simulink model "Nerthus_sim"  (R2022a)
settings: Solver=ode45  StartTime=0.0  StopTime=simtime  FixedStep=0.1  MaxStep=0.1
values from neighbouring files (symbols this model uses):
  a_f = (1E-5)*depl_fuel_temp_coef(depl_index)    [parameters.m]
  a_g = 1E-5*depl_grap_temp_coef(depl_index)    [parameters.m]
  A_s = 1.2245    [parameters.m]
  beta = depl_beta(depl_index,:)    [parameters.m]
  beta_t = sum(beta)    [parameters.m]
  Cp_1 = mean(interp1(Cal_temp1, Cal_Cp1, region_fdw))/1e3    [parameters.m]
  Cp_2 = mean(interp1(Cal_temp2, Cal_Cp2, region_sc))/1e3    [parameters.m]
  Cp_3 = mean(interp1(Cal_temp3, Cal_Cp3, region_s2))/1e3    [parameters.m]
  Cp_4 = mean(interp1(Cal_temp4, Cal_Cp4, region_s1))/1e3    [parameters.m]
  Cp_p = 0.00154912    [parameters.m]
  Cp_w = 456.056e-6    (= 0.000456056)    [parameters.m]
  D_it = 0.0141478    [parameters.m]
  D_ot = 0.015875    [parameters.m]
  DHRS_MODE = 2    [ColdSlug.m]    (also in ReactivityInsertion.m = 1; ULOF.m = 1; transients.m = 1)
  DHRS_Power = P*(0.10)    (= 55.7)    [ColdSlug.m]    (also in ReactivityInsertion.m; ULOF.m; transients.m)
  DHRS_time = 2000    [ColdSlug.m]    (also in ReactivityInsertion.m = 2000000; ULOF.m; transients.m = 2000000)
  DHRS_TIME_K = 10    [parameters.m]
  dHs_dPs = -0.042433622114357    (= -0.0424336221144)    [parameters.m]
  Epsilon = 1E-3    (= 0.001)    [parameters.m]
  Fiss_factor = 2.464783802008740e-03    (= 0.00246478380201)    [parameters.m]
  gamma0 = 9.635981959409105e-01    (= 0.963598195941)    [parameters.m]
  gamma1 = 3.560674858154914e-02    (= 0.0356067485815)    [parameters.m]
  gamma2 = 7.950554775404400e-04    (= 0.00079505547754)    [parameters.m]
  gamma_I = 5.1135e-2    (= 0.051135)    [parameters.m]
  gamma_Te = 6.1e-2    (= 0.061)    [parameters.m]
  gamma_Xe = 1.1628e-2    (= 0.011628)    [parameters.m]
  h_pw = h_s_shx    (= 0.00910134357894)    [parameters.m]
  H_s_table = zeros(m, n)    [parameters.m]
  h_wb = 13349.334646671E-6    (= 0.0133493346467)    [parameters.m]
  h_ws = 5732.378387768E-6    (= 0.00573237838777)    [parameters.m]
  h_wsc = 8385.005556375E-6    (= 0.00838500555638)    [parameters.m]
  hA_fg = (12.5325)*SF_area_CORE    [parameters.m]
  hA_p_phx1 = [UA_phx_nm,UA_phx_nm,UA_phx_nm,UA_phx_nm]    [parameters.m]
  hA_p_shx1 = [UA_shx_nm,UA_shx_nm,UA_shx_nm,UA_shx_nm]    [parameters.m]
  hA_s_phx1 = [UA_phx_nm,UA_phx_nm,UA_phx_nm,UA_phx_nm]    [parameters.m]
  hA_s_shx1 = [UA_shx_nm,UA_shx_nm,UA_shx_nm,UA_shx_nm]    [parameters.m]
  I_0 = ((gamma_I*Sig_f*phi_0) + (lam_Te*Te_0))/lam_I    (= 1.07253115949e+22)    [parameters.m]
  k_1 = 0.5    [parameters.m]
  K_1 = 11.632248097704855    (= 11.6322480977)    [parameters.m]
  k_2 = 0.5    [parameters.m]
  K_4 = b(1)    [parameters.m]
  K_5 = a(1)    [parameters.m]
  K_b = 12.834854076292217    (= 12.8348540763)    [parameters.m]
  k_f1 = k_f/nn_f    (= 0.465)    [parameters.m]
  k_f2 = k_f/nn_f    (= 0.465)    [parameters.m]
  k_g = 0.07    [parameters.m]
  K_pump = 0.2    [parameters.m]
  K_sc = -17.615718797133468    (= -17.6157187971)    [parameters.m]
  L = 8.5344*SF_length    [parameters.m]
  L_b = 2.3645*SF_length    [parameters.m]
  L_s = 4.723*SF_length    [parameters.m]
  L_sc = 1.4469*SF_length    [parameters.m]
  Lam = depl_Lam(depl_index)    [parameters.m]
  lam = [1.240E-02, 3.05E-02, 1.11E-01, 3.01E-01, 1.140E+00, 3.014E+00]    [parameters.m]
  lam_bubl = 0.0    (= 0)    [parameters.m]
  lam_I = 2.875e-5    (= 2.875e-05)    [parameters.m]
  lam_Te = 3.65e-02    (= 0.0365)    [parameters.m]
  lam_Xe = 2.0916e-5    (= 2.0916e-05)    [parameters.m]
  lambda0 = 0.0945298    [parameters.m]
  lambda1 = 0.00441957    [parameters.m]
  lambda2 = 8.60979e-05    [parameters.m]
  m_f_t = mdot_fuel*(tau_core + tau_phx + tau_DHRS)    [parameters.m]
  M_initial = L_b*rho_b*A_s + L_s*rho_s*A_s + L_sc*A_s*rho_sc    [parameters.m]
  M_stm = 0.018    [parameters.m]
  mcp_f1 = mn_f*scp_fuel    [parameters.m]
  mcp_f2 = mn_f*scp_fuel    [parameters.m]
  mcp_g1 = m_g*scp_graphite    [parameters.m]
  mcp_p_phx1 = scp_fuel*mp_phx1    [parameters.m]
  mcp_p_shx1 = scp_coolant*mp_shx1    [parameters.m]
  mcp_s_phx1 = scp_coolant*ms_phx1    [parameters.m]
  mcp_s_shx1 = scp_HITEC*ms_shx1    [parameters.m]
  mcp_t_phx1 = scp_tube*mt_phx1    [parameters.m]
  mcp_t_shx1 = scp_tube*mt_shx1    [parameters.m]
  mdot_coolant = 1543 + SF_fdw_PHX    [parameters.m]
  mdot_HITEC = 3379 + SF_fdw_SHX    [parameters.m]
  mn_f = (m_f/nn_f)    [parameters.m]
  mn_piDHRS = mdot_fuel*tau_DHRS    [parameters.m]
  mn_UHX = (tau_HITEC_UHX*mdot_HITEC)/n_UHX    [parameters.m]
  mp_phx1 = [mp_phx_nm, mp_phx_nm, mp_phx_nm, mp_phx_nm]    [parameters.m]
  mp_shx1 = [mp_shx_nm, mp_shx_nm, mp_shx_nm, mp_shx_nm]    [parameters.m]
  ms_phx1 = [ms_phx_nm, ms_phx_nm, ms_phx_nm, ms_phx_nm]    [parameters.m]
  ms_shx1 = [ms_shx_nm, ms_shx_nm, ms_shx_nm, ms_shx_nm]    [parameters.m]
  N = 6546*SF_linear    [parameters.m]    (also in plot_better.m = load('Results\Core_Out_TempA2.mat'))
  n_frac0 = 1    [parameters.m]
  n_UHX = 3    [parameters.m]
  omega = 10.00000    (= 10)    [ColdSlug.m]    (also in ReactivityInsertion.m; ULOF.m; transients.m)
  P = 557    [ColdSlug.m]    (also in ReactivityInsertion.m; ULOF.m; plot_better.m = load('Results\Total_Power2.mat'); transients.m)
  P_s = 12.5    [parameters.m]
  P_sat = 12.5    [parameters.m]
  P_sc = 12.5    [parameters.m]
  phi_0 = 2.00819E+22    (= 2.00819e+22)    [parameters.m]
  Power_Bleed = P*(0.00)    (= 0)    [ColdSlug.m]    (also in ReactivityInsertion.m; ULOF.m; parameters.m = P*(0.01); transients.m)
  pres_table = pres_inp    [parameters.m]
  R = 8.314462E-6    (= 8.314462e-06)    [parameters.m]
  rho_0 = beta_t - bterm    [parameters.m]
  rho_b = (XSteam('rho_pT', 125, 327.81) + XSteam('rho_pT', 125, 327.82))/2    [parameters.m]
  rho_p = rho_HITEC    (= 1680)    [parameters.m]
  rho_s = mean(interp1(Cal_temp_steam, Cal_rho3, region_steam))    [parameters.m]
  rho_sc = mean(interp1(Cal_temp2, Cal_rho2, region_sc))    [parameters.m]
  rho_w = 8425.712    [parameters.m]
  rhoXe_0 = (-sig_Xe / Sig_a) * (gamma_Te + gamma_I + gamma_Xe) * Sig_f * phi_0/(lam_Xe + sig_Xe * phi_0 + lam_bubl)    (= -0.0117027857895)    [parameters.m]
  scp_coolant = 8.83E-3    (= 0.00883)    [parameters.m]
  scp_fuel = 1.9665E-3    (= 0.0019665)    [parameters.m]
  scp_HITEC = 0.00154912    [parameters.m]
  Sig_f = 1.36931e-4    (= 0.000136931)    [parameters.m]
  sig_Xe = 2.66449e-18    [parameters.m]
  sin_mag = 0    [ColdSlug.m]    (also in ReactivityInsertion.m; ULOF.m; transients.m)
  T0_f1 = Tf_in + (T0_f2-Tf_in)/2    (= 649.2)    [parameters.m]
  T0_f2 = 681.8    [parameters.m]
  T0_g1 = T0_f1 + (k_g*P/hA_fg)    [parameters.m]
  T0_p_phx1 = [663.1, 644.3, 630.3, 616.6]    [parameters.m]
  T0_p_shx1 = [641.8, 656.3, 621.4, 586.4]    [parameters.m]
  T0_s_phx1 = [595.1, 603.8, 615.6, 627.3]    [parameters.m]
  T0_s_shx1 = [598.2, 689.1, 651.4, 613.7]    [parameters.m]
  T0_t_phx1 = [639.3, 612.7]    [parameters.m]
  T0_t_shx1 = [646.6, 609.8]    [parameters.m]
  T_fw = 180.0    (= 180)    [parameters.m]
  T_p1 = 605.5    [parameters.m]
  T_p2 = 579.6    [parameters.m]
  T_p3 = 557.5    [parameters.m]
  ... (+40 more)
undefined symbols (not defined in the file or in its folder): C0, Cp_s, Cp_sc, ln, rho_f, scp_f, scp_s, Sig_f_msdr, vdot_f, vdot_s
libraries: slpidlib x1, simulink x1
(part 3 of 3)

== system Nerthus_sim/TEST BLOCKS/Primary loop constant heat removal ==
  In1 : Inport
  Fcn : Fcn  Expr=u(1) - P/(vdot_f*rho_f*scp_f)
  Mux : Mux  Inputs=2
  Out1 : Outport  VectorParamsAs1DForOutWhenUnconnected=off
  wires:
  In1/1 -> Mux/1
  Fcn/1 -> Out1/1, Mux/2
  Mux/1 -> Fcn/1

== system Nerthus_sim/TEST BLOCKS/Secondaary loop constant heat production ==
  In1 : Inport
  Fcn : Fcn  Expr=u(1) + P/(vdot_s*rho_s*scp_s)
  Mux : Mux  Inputs=2
  Out1 : Outport  VectorParamsAs1DForOutWhenUnconnected=off
  wires:
  In1/1 -> Mux/1
  Fcn/1 -> Out1/1, Mux/2
  Mux/1 -> Fcn/1

== system Nerthus_sim/TEST BLOCKS/Secondary loop constant heat removal ==
  In1 : Inport
  Fcn : Fcn  Expr=u(1) - P/(vdot_s*rho_s*scp_s)
  Mux : Mux  Inputs=2
  Out1 : Outport  VectorParamsAs1DForOutWhenUnconnected=off
  wires:
  In1/1 -> Mux/1
  Fcn/1 -> Out1/1, Mux/2
  Mux/1 -> Fcn/1

== system Nerthus_sim/UHX/UHX ==
  HITEC_INLET : Inport
  HITEC_FLOW_FRAC : Inport  Port=2
  Enable : EnablePort
  Demand From Workspace : FromWorkspace  VariableName=demand  SampleTime=1  Interpolate=off  OutputAfterFinalValue=Holding final value
  Mux2 : Mux  Inputs=6
      settings: DisplayOption=signals
  Tp1_otsg : Integrator  InitialCondition=T0_s_shx1(1)
  Tp2_otsg : Integrator  InitialCondition=T0_s_shx1(1)
  Tp3_otsg : Integrator  InitialCondition=T0_s_shx1(1)
  d(Tp1_UHX)/dt : Fcn  Expr=(u[2]*mdot_HITEC/mn_UHX)*(u[1]-u[4]) - (u[3]*P/n_UHX)/(mn_UHX*scp_HITEC)
  d(Tp2_UHX)/dt : Fcn  Expr=(u[2]*mdot_HITEC/mn_UHX)*(u[4]-u[5]) - (u[3]*P/n_UHX)/(mn_UHX*scp_HITEC)
  d(Tp3_UHX)/dt : Fcn  Expr=(u[2]*mdot_HITEC/mn_UHX)*(u[5]-u[6]) - (u[3]*P/n_UHX)/(mn_UHX*scp_HITEC)
  HITEC_OUTLET : Outport  VectorParamsAs1DForOutWhenUnconnected=off
  wires:
  Tp2_otsg/1 -> Mux2/5
  HITEC_INLET/1 -> Mux2/1
  Mux2/1 -> d(Tp1_UHX)/dt/1, d(Tp2_UHX)/dt/1, d(Tp3_UHX)/dt/1
  d(Tp1_UHX)/dt/1 -> Tp1_otsg/1
  d(Tp2_UHX)/dt/1 -> Tp2_otsg/1
  d(Tp3_UHX)/dt/1 -> Tp3_otsg/1
  Demand From Workspace/1 -> Mux2/3
  HITEC_FLOW_FRAC/1 -> Mux2/2
  Tp1_otsg/1 -> Mux2/4
  Tp3_otsg/1 -> HITEC_OUTLET/1, Mux2/6

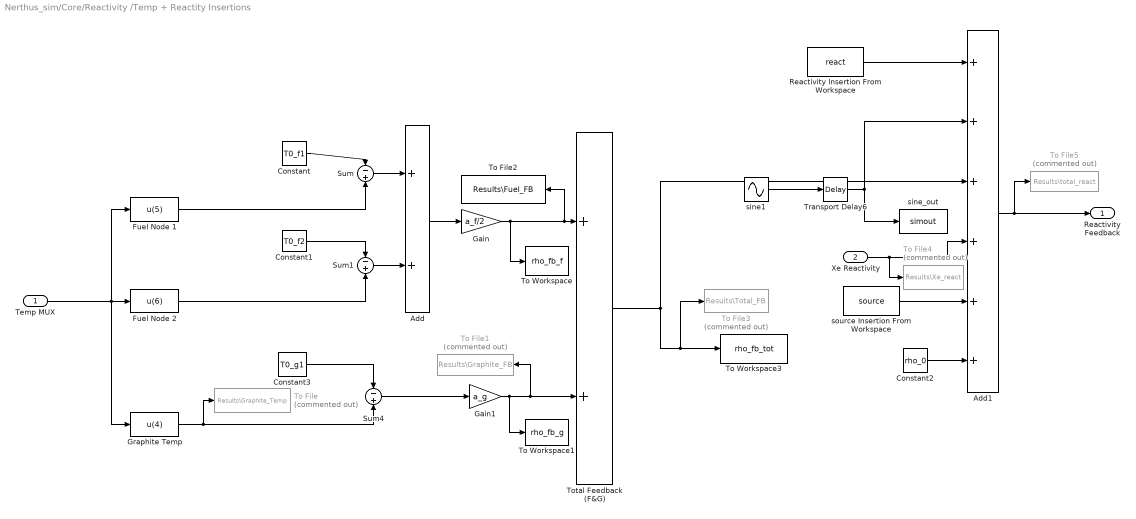
== system Nerthus_sim/Core/Reactivity /Temp + Reactity Insertions ==
  "Temp MUX " : Inport
  Xe Reactivity : Inport  Port=2
  Add : Sum
  Add1 : Sum  Inputs=++++++
  Constant : Constant  Value=T0_f1
  Constant1 : Constant  Value=T0_f2
  Constant2 : Constant  Value=rho_0
  Constant3 : Constant  Value=T0_g1
  "Fuel Node 1 " : Fcn  Expr=u(5)
  Fuel Node 2 : Fcn  Expr=u(6)
  Gain : Gain  Gain=a_f/2
  Gain1 : Gain  Gain=a_g
  Graphite Temp : Fcn  Expr=u(4)
  Reactivity Insertion From Workspace : FromWorkspace  VariableName=react  SampleTime=1  Interpolate=off  OutputAfterFinalValue=Holding final value
  Sum : Sum  Inputs=-|+
  Sum1 : Sum  Inputs=-|+
  Sum4 : Sum  Inputs=-|+
  To File : ToFile  Commented=on  Filename=Results\Graphite_Temp  MatrixName=Graphite_Temp
  To File1 : ToFile  Commented=on  Filename=Results\Graphite_FB  MatrixName=Graphite_FB
  To File2 : ToFile  Filename=Results\Fuel_FB  MatrixName=Fuel_FB
  To File3 : ToFile  Commented=on  Filename=Results\Total_FB  MatrixName=Total_FB
  To File4 : ToFile  Commented=on  Filename=Results\Xe_react  MatrixName=Xe_react
  To File5 : ToFile  Commented=on  Filename=Results\total_react  MatrixName=total_react
  To Workspace : ToWorkspace  VariableName=rho_fb_f  SampleTime=-1
  To Workspace1 : ToWorkspace  VariableName=rho_fb_g  SampleTime=-1
  To Workspace3 : ToWorkspace  VariableName=rho_fb_tot  SampleTime=-1
  Total Feedback (F&G) : Sum
  Transport Delay6 : TransportDelay  DelayTime=1000  BufferSize=4096
  sine1 : Sin  Amplitude=sin_mag  Frequency=omega  SampleTime=0
  sine_out : ToWorkspace  VariableName=simout  SampleTime=-1
  source Insertion From Workspace : FromWorkspace  VariableName=source  SampleTime=1  Interpolate=off  OutputAfterFinalValue=Holding final value
  Reactivity Feedback : Outport  VectorParamsAs1DForOutWhenUnconnected=off
  wires:
  Constant3/1 -> Sum4/1
  Sum/1 -> Add/1
  Add1/1 -> To File5/1, Reactivity Feedback/1
  Gain1/1 -> To Workspace1/1, To File1/1, Total Feedback (F&G)/2
  "Fuel Node 1 "/1 -> Sum/2
  Reactivity Insertion From Workspace/1 -> Add1/1
  Add/1 -> Gain/1
  Total Feedback (F&G)/1 -> To File3/1, To Workspace3/1, Add1/3
  Sum1/1 -> Add/2
  Graphite Temp/1 -> To File/1, Sum4/2
  Constant1/1 -> Sum1/1
  Sum4/1 -> Gain1/1
  Constant/1 -> Sum/1
  Transport Delay6/1 -> sine_out/1, Add1/2
  Gain/1 -> To Workspace/1, To File2/1, Total Feedback (F&G)/1
  sine1/1 -> Transport Delay6/1
  Fuel Node 2/1 -> Sum1/2
  Xe Reactivity/1 -> Add1/4, To File4/1
  source Insertion From Workspace/1 -> Add1/5
  Constant2/1 -> Add1/6
  "Temp MUX "/1 -> "Fuel Node 1 "/1, Graphite Temp/1, Fuel Node 2/1

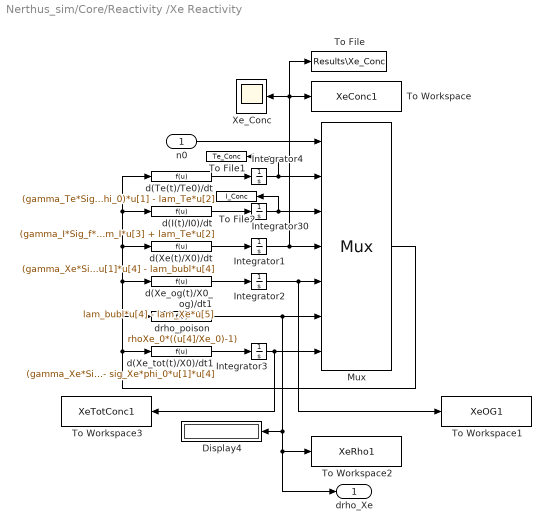
== system Nerthus_sim/Core/Reactivity /Xe Reactivity ==
  n0 : Inport
  Display4 : Display
  Integrator1 : Integrator  InitialCondition=Xe_0
  Integrator2 : Integrator  InitialCondition=Xe_og
  Integrator3 : Integrator  InitialCondition=Xe_0+Xe_og
  Integrator30 : Integrator  InitialCondition=I_0
  Integrator4 : Integrator  InitialCondition=Te_0
  Mux : Mux  Inputs=7
      settings: DisplayOption=signals
  To File : ToFile  Filename=Results\Xe_Conc  MatrixName=Xe_Conc
  To File1 : ToFile  Filename=Te_Conc  MatrixName=Te_Conc
  To File2 : ToFile  Filename=I_Conc  MatrixName=I_Conc
  To Workspace : ToWorkspace  VariableName=XeConc1  SampleTime=-1
  To Workspace1 : ToWorkspace  VariableName=XeOG1  SampleTime=-1
  To Workspace2 : ToWorkspace  VariableName=XeRho1  SampleTime=-1
  To Workspace3 : ToWorkspace  VariableName=XeTotConc1  SampleTime=-1
  Xe_Conc : Scope
  d(I(t)/I0)/dt : Fcn  Expr=(gamma_I*Sig_f*phi_0)*u[1] - lam_I*u[3] + lam_Te*u[2]
  d(Te(t)/Te0)/dt : Fcn  Expr=(gamma_Te*Sig_f*phi_0)*u[1] - lam_Te*u[2]
  d(Xe(t)/X0)/dt : Fcn  Expr=(gamma_Xe*Sig_f*phi_0)*u[1] + lam_I*u[3] - lam_Xe*u[4] - sig_Xe*phi_0*u[1]*u[4] - lam_bubl*u[4]
  d(Xe_og(t)/X0_og)/dt1 : Fcn  Expr=lam_bubl*u[4] - lam_Xe*u[5]
  d(Xe_tot(t)/X0)/dt1 : Fcn  Expr=(gamma_Xe*Sig_f*phi_0)*u[1] + lam_I*u[3] - lam_Xe*u[4] - sig_Xe*phi_0*u[1]*u[4]
  drho_poison : Fcn  Expr=rhoXe_0*((u[4]/Xe_0)-1)
  drho_Xe : Outport  VectorParamsAs1DForOutWhenUnconnected=off
  wires:
  Integrator2/1 -> To Workspace1/1, Mux/5
  n0/1 -> Mux/1
  d(I(t)/I0)/dt/1 -> Integrator30/1
  Integrator30/1 -> To File2/1, Mux/3
  Integrator3/1 -> Mux/7, To Workspace3/1
  drho_poison/1 -> Display4/1, To Workspace2/1, drho_Xe/1, Mux/6
  d(Xe_og(t)/X0_og)/dt1/1 -> Integrator2/1
  Integrator1/1 -> To File/1, Xe_Conc/1, To Workspace/1, Mux/4
  d(Xe(t)/X0)/dt/1 -> Integrator1/1
  Integrator4/1 -> To File1/1, Mux/2
  d(Te(t)/Te0)/dt/1 -> Integrator4/1
  d(Xe_tot(t)/X0)/dt1/1 -> Integrator3/1
  Mux/1 -> d(Xe_og(t)/X0_og)/dt1/1, d(Te(t)/Te0)/dt/1, d(I(t)/I0)/dt/1, d(Xe(t)/X0)/dt/1, drho_poison/1, d(Xe_tot(t)/X0)/dt1/1

== system Nerthus_sim/Core/Reactivity /Xe Reactivity Old ==
  n0 : Inport
  Integrator1 : Integrator  InitialCondition=Xe_0
  Integrator2 : Integrator  InitialCondition=Xe_og
  Integrator30 : Integrator  InitialCondition=I_0
  Mux : Mux  Inputs=5
      settings: DisplayOption=signals
  Unit Delay : UnitDelay  SampleTime=-1  HasFrameUpgradeWarning=on
  d(I(t)/I0)/dt : Fcn  Expr=(gamma_I*Sig_f_msdr*phi_0)*u[1] - lam_I*u[2]
  d(Xe(t)/X0)/dt : Fcn  Expr=(gamma_Xe*Sig_f_msdr*phi_0)*u[1] + lam_I*u[2] - lam_Xe*u[3] - sig_Xe*phi_0*u[1]*u[3] - lam_bubl*u[3]
  d(Xe_og(t)/X0_og)/dt1 : Fcn  Expr=lam_bubl*u[3] - lam_Xe*u[4]
  drho_poison : Fcn  Expr=rhoXe_0*((u[3]/Xe_0)-1)
  drho_Xe : Outport  VectorParamsAs1DForOutWhenUnconnected=off
  wires:
  Integrator1/1 -> Mux/3
  Mux/1 -> d(Xe_og(t)/X0_og)/dt1/1, d(I(t)/I0)/dt/1, d(Xe(t)/X0)/dt/1, drho_poison/1
  Integrator2/1 -> Mux/4
  Unit Delay/1 -> Mux/5, drho_Xe/1
  n0/1 -> Mux/1
  drho_poison/1 -> Unit Delay/1
  d(Xe(t)/X0)/dt/1 -> Integrator1/1
  Integrator30/1 -> Mux/2
  d(Xe_og(t)/X0_og)/dt1/1 -> Integrator2/1
  d(I(t)/I0)/dt/1 -> Integrator30/1

== system Nerthus_sim/Core/Reactivity /Xe Reactivity1 ==
  n0 : Inport
  Integrator1 : Integrator  InitialCondition=Xe_0
  Integrator2 : Integrator  InitialCondition=Xe_og
  Integrator3 : Integrator  InitialCondition=Xe_0+Xe_og
  Integrator30 : Integrator  InitialCondition=I_0
  Mux : Mux  Inputs=6
      settings: DisplayOption=signals
  To Workspace : ToWorkspace  VariableName=XeConc  SampleTime=-1
  To Workspace1 : ToWorkspace  VariableName=XeOG  SampleTime=-1
  To Workspace2 : ToWorkspace  VariableName=XeRho  SampleTime=-1
  To Workspace3 : ToWorkspace  VariableName=XeTotConc  SampleTime=-1
  d(I(t)/I0)/dt : Fcn  Expr=(gamma_I*Sig_f_msdr*phi_0)*u[1] - lam_I*u[2]
  d(Xe(t)/X0)/dt : Fcn  Expr=(gamma_Xe*Sig_f_msdr*phi_0)*u[1] + lam_I*u[2] - lam_Xe*u[3] - sig_Xe*phi_0*u[1]*u[3] - lam_bubl*u[3]
  d(Xe_og(t)/X0_og)/dt1 : Fcn  Expr=lam_bubl*u[3] - lam_Xe*u[4]
  d(Xe_tot(t)/X0)/dt1 : Fcn  Expr=(gamma_Xe*Sig_f_msdr*phi_0)*u[1] + lam_I*u[2] - lam_Xe*u[3] - sig_Xe*phi_0*u[1]*u[3]
  drho_poison : Fcn  Expr=rhoXe_0*((u[3]/Xe_0)-1)
  drho_Xe : Outport  VectorParamsAs1DForOutWhenUnconnected=off
  wires:
  Integrator3/1 -> Mux/6, To Workspace3/1
  d(Xe_tot(t)/X0)/dt1/1 -> Integrator3/1
  d(I(t)/I0)/dt/1 -> Integrator30/1
  d(Xe_og(t)/X0_og)/dt1/1 -> Integrator2/1
  Integrator30/1 -> Mux/2
  d(Xe(t)/X0)/dt/1 -> Integrator1/1
  n0/1 -> Mux/1
  drho_poison/1 -> drho_Xe/1, To Workspace2/1, Mux/5
  Integrator2/1 -> Mux/4, To Workspace1/1
  Mux/1 -> d(Xe_tot(t)/X0)/dt1/1, drho_poison/1, d(Xe(t)/X0)/dt/1, d(I(t)/I0)/dt/1, d(Xe_og(t)/X0_og)/dt1/1
  Integrator1/1 -> Mux/3, To Workspace/1
